simulink model "torque_control_model_7"  (R2018b)
settings: Solver=VariableStepAuto  StartTime=0.0  StopTime=.5  RelTol=1e-3
PreLoadFcn:
  | BLDC_motor_constants_2;
undefined symbols (not defined in the file or in its folder): sigbuilder_block
libraries: powerlib x13, simulink x2, peBldcCurrentController x1
settings Model: Creator=Zach  LastModifiedBy=Zach

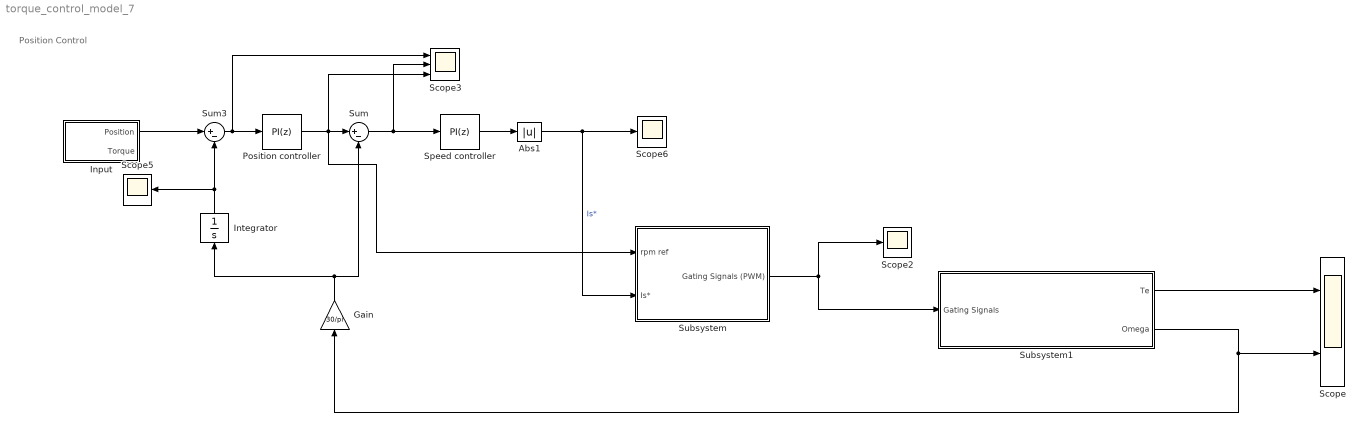
== system torque_control_model_7 ==
  note: Position Control
  Abs1 : Abs
  Gain : Gain  Gain=30/pi
  Input : Subsystem  Tag=STV Subsys  LoadFcn=sigbuilder_block('load');  StartFcn=sigbuilder_block('start');  StopFcn=sigbuilder_block('stop');  ClipboardFcn=sigbuilder_block('clipboard');  mask(Sigbuilder block){tuvar=[0:10]}
      mask help: Simulink:masks:SigbuilderBlock_MD
      mask init:
      | if ~strcmp(get_param(bdroot(gcbh),'SimulationStatus'),'stopped') tuvar = sigbuilder_block('maskInit'); end
      settings: CopyFcn=sigbuilder_block('copy');  DeleteFcn=sigbuilder_block('delete');  ModelCloseFcn=sigbuilder_block('modelClose');  PreSaveFcn=sigbuilder_block('preSave');  PauseFcn=sigbuilder_block('pause');  ContinueFcn=sigbuilder_block('continue');  NameChangeFcn=sigbuilder_block('namechange');  OpenFcn=sigbuilder_block('open',[268.5 149.25 631.5 540 ]);  CloseFcn=sigbuilder_block('close');
      mask Display: plot(0, 0, 100, 100,[2, 2, 32, 32, 2], [68, 8, 8, 68, 68],[32, 2], [38, 38], [32, 19, 2],[53, 60, 44], [32, 17, 17, 2],[16, 16, 31, 31]);txt = getActiveGroup(gcbh);text(2, 100, txt,'verticalAlignment', 'top');
  Integrator : Integrator
  Position controller : simulink/Continuous/PID Controller  Controller=PI  Form=Parallel  TimeDomain=Discrete-time  SampleTime=-1  IntegratorMethod=Forward Euler  FilterMethod=Forward Euler  ControllerParametersSource=internal  P=80  I=5  D=0.5  UseFilter=on  N=100  TunerSelectOption=Transfer Function Based (PID Tuner App)  InitialConditionSource=internal  InitialConditionForIntegrator=0  InitialConditionForFilter=0  DifferentiatorICPrevScaledInput=0  ExternalReset=none  TrackingMode=off  Kt=1  LimitOutput=off  UpperSaturationLimit=10000  LowerSaturationLimit=-10000  LinearizeAsGain=on  AntiWindupMode=back-calculation  Kb=100  POutMin=[]  POutMax=[]  IOutMin=[]  IOutMax=[]  DOutMin=[]  DOutMax=[]  NOutMin=[]  NOutMax=[]  SumOutMin=[]  SumOutMax=[]  SaturationOutMin=[]  SaturationOutMax=[]  PParamMin=[]  PParamMax=[]  IParamMin=[]  IParamMax=[]  DParamMin=[]  DParamMax=[]  NParamMin=[]  NParamMax=[]  KbParamMin=[]  KbParamMax=[]  KtParamMin=[]  KtParamMax=[]  KbOutMin=[]  KbOutMax=[]  KtOutMin=[]  KtOutMax=[]  IntegratorOutMin=[]  IntegratorOutMax=[]  FilterOutMin=[]  FilterOutMax=[]  SumI1OutMin=[]  SumI1OutMax=[]  SumI2OutMin=[]  SumI2OutMax=[]  SumI3OutMin=[]  SumI3OutMax=[]  SumI4OutMin=[]  SumI4OutMax=[]  SumDOutMin=[]  SumDOutMax=[]  DifferentiatorOutMin=[]  DifferentiatorOutMax=[]  FilterDiffOutCoefMin=[]  FilterDiffOutCoefMax=[]  ReciprocalOutMin=[]  ReciprocalOutMax=[]  SumDenOutMin=[]  SumDenOutMax=[]  SumNumOutMin=[]  SumNumOutMax=[]  DivideOutMin=[]  DivideOutMax=[]  IntegratorContinuousStateAttributes=''  IntegratorStateMustResolveToSignalObject=off  IntegratorRTWStateStorageClass=Auto  FilterContinuousStateAttributes=''  FilterStateMustResolveToSignalObject=off  FilterRTWStateStorageClass=Auto  ParallelPVariant=InternalParameters  IdealPVariant=Disabled  IVariant=InternalParameters  DVariant=Disabled  IntegratorVariant=Discrete  SatVariant=Disabled  AWVariant=Passthrough  PCopyVariant=Disabled  TRVariant=Disabled  FdbkBlocksVariant=Forward  IdealPFdbkVariant=Disabled  SatFdbkVariant=Disabled  DerivativeFilterVariant=Disabled  NVariant=Disabled  NCopyVariant=Disabled_SignalSpec  FilterICVariant=Disabled  IntegratorICVariant=InternalICs  ExternalResetVariant=Disabled  TRSumVariant=Passthrough  SumFdbkVariant=Disabled  SumVariant=Sum_PI
  Scope : Scope  NumInputPorts=2
  Scope2 : Scope
  Scope3 : Scope  NumInputPorts=3
  Scope5 : Scope
  Scope6 : Scope
  Speed controller : simulink/Continuous/PID Controller  Controller=PI  Form=Parallel  TimeDomain=Discrete-time  SampleTime=-1  IntegratorMethod=Forward Euler  FilterMethod=Forward Euler  ControllerParametersSource=internal  P=.01  I=15  D=0.5  UseFilter=on  N=100  TunerSelectOption=Transfer Function Based (PID Tuner App)  InitialConditionSource=internal  InitialConditionForIntegrator=0  InitialConditionForFilter=0  DifferentiatorICPrevScaledInput=0  ExternalReset=none  TrackingMode=off  Kt=1  LimitOutput=on  UpperSaturationLimit=500  LowerSaturationLimit=-500  LinearizeAsGain=on  AntiWindupMode=back-calculation  Kb=100  POutMin=[]  POutMax=[]  IOutMin=[]  IOutMax=[]  DOutMin=[]  DOutMax=[]  NOutMin=[]  NOutMax=[]  SumOutMin=[]  SumOutMax=[]  SaturationOutMin=[]  SaturationOutMax=[]  PParamMin=[]  PParamMax=[]  IParamMin=[]  IParamMax=[]  DParamMin=[]  DParamMax=[]  NParamMin=[]  NParamMax=[]  KbParamMin=[]  KbParamMax=[]  KtParamMin=[]  KtParamMax=[]  KbOutMin=[]  KbOutMax=[]  KtOutMin=[]  KtOutMax=[]  IntegratorOutMin=[]  IntegratorOutMax=[]  FilterOutMin=[]  FilterOutMax=[]  SumI1OutMin=[]  SumI1OutMax=[]  SumI2OutMin=[]  SumI2OutMax=[]  SumI3OutMin=[]  SumI3OutMax=[]  SumI4OutMin=[]  SumI4OutMax=[]  SumDOutMin=[]  SumDOutMax=[]  DifferentiatorOutMin=[]  DifferentiatorOutMax=[]  FilterDiffOutCoefMin=[]  FilterDiffOutCoefMax=[]  ReciprocalOutMin=[]  ReciprocalOutMax=[]  SumDenOutMin=[]  SumDenOutMax=[]  SumNumOutMin=[]  SumNumOutMax=[]  DivideOutMin=[]  DivideOutMax=[]  IntegratorContinuousStateAttributes=''  IntegratorStateMustResolveToSignalObject=off  IntegratorRTWStateStorageClass=Auto  FilterContinuousStateAttributes=''  FilterStateMustResolveToSignalObject=off  FilterRTWStateStorageClass=Auto  ParallelPVariant=InternalParameters  IdealPVariant=Disabled  IVariant=InternalParameters  DVariant=Disabled  IntegratorVariant=Discrete  SatVariant=Enabled  AWVariant=BackCalculation  PCopyVariant=Disabled  TRVariant=Disabled  FdbkBlocksVariant=Forward  IdealPFdbkVariant=Disabled  SatFdbkVariant=Disabled  DerivativeFilterVariant=Disabled  NVariant=Disabled  NCopyVariant=Disabled_SignalSpec  FilterICVariant=Disabled  IntegratorICVariant=InternalICs  ExternalResetVariant=Disabled  TRSumVariant=Passthrough  SumFdbkVariant=Disabled  SumVariant=Sum_PI
  Subsystem : Subsystem
  Subsystem1 : Subsystem
  Sum : Sum  Inputs=|+-
  Sum3 : Sum  Inputs=|+-
  wires:
  Subsystem1/1(Te) -> Scope/1
  Position controller/1 -> Subsystem/1(rpm ref), Sum/1, Scope3/3
  Speed controller/1 -> Abs1/1
  Sum/1 -> Scope3/2, Speed controller/1
  Subsystem1/2(Omega) -> Scope/2, Gain/1
  Sum3/1 -> Scope3/1, Position controller/1
  Integrator/1 -> Sum3/2, Scope5/1
  Input/1(Position) -> Sum3/1
  Abs1/1 -> Scope6/1, Subsystem/2(Is*)  "Is*"
  Gain/1 -> Integrator/1, Sum/2
  Subsystem/1(Gating Signals (PWM)) -> Subsystem1/1(Gating Signals), Scope2/1

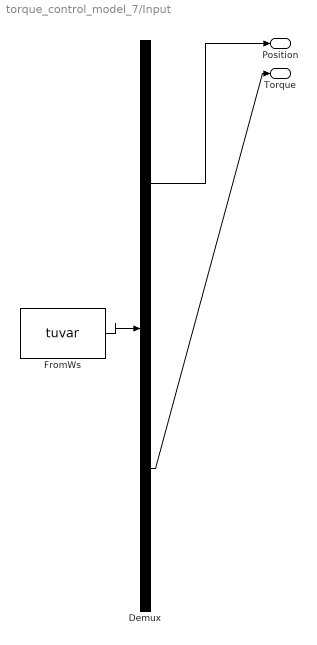
== system torque_control_model_7/Input ==
  Demux : Demux  Tag=STV Demux  Outputs=2
  FromWs : FromWorkspace  Tag=STV FromWs  VariableName=tuvar  SampleTime=0
      SigBuilderData=|
      | common.afterFinalStr = 'Extrapolate'
      | common.sampleTime = 0
      | dataSet.timeRange = [0 2]
      | dataSet.name = 'Test 1'
      | sbobj.Groups.Name = 'Test 1'
      | sbobj.Groups.Signals(1).Name = 'Position'
      | sbobj.Groups.Signals(1).XData = [0 0.1 0.1 0.805 0.805 1.405 1.405 2]
      | sbobj.Groups.Signals(1).YData = [0 1 80 80 100 100 20 20]
      | sbobj.Groups.Signals(2).Name = 'Torque'
      | sbobj.Groups.Signals(2).XData = [0 0.5 0.5 2]
      | sbobj.Groups.Signals(2).YData = [0 0 3 3]
      | sbobj.Groups.TimeRange = [0 2]
  Position : Outport  Tag=STV Outport
  Torque : Outport  Tag=STV Outport  Port=2
  wires:
  FromWs/1 -> Demux/1
  Demux/1 -> Position/1
  Demux/2 -> Torque/1

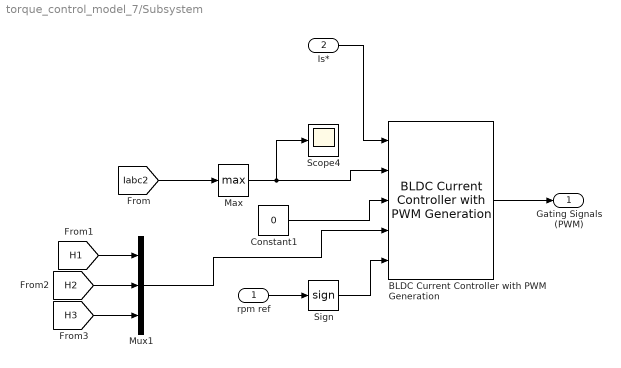
== system torque_control_model_7/Subsystem ==
  rpm ref : Inport
  Is* : Inport  Port=2
  BLDC Current Controller with PWM Generation : peBldcCurrentController/BLDC Current Controller with PWM Generation  Kp=40  Ki=1  Kaw=100  Ts=-1  Tsd=0.001  ActZC=off  CarrCount=Up  Tper=.0001  Tfundamental=.00001
  Constant1 : Constant  Value=0
  Max : MinMax  Function=max
  Mux1 : Mux  Inputs=3
  Scope4 : Scope
  Sign : Signum
  Gating Signals (PWM) : Outport
  wires:
  rpm ref/1 -> Sign/1
  Mux1/1 -> BLDC Current Controller with PWM Generation/4
  [Iabc2] -> Max/1
  [H1] -> Mux1/1
  [H3] -> Mux1/3
  Sign/1 -> BLDC Current Controller with PWM Generation/5
  Constant1/1 -> BLDC Current Controller with PWM Generation/3
  Max/1 -> BLDC Current Controller with PWM Generation/2, Scope4/1
  [H2] -> Mux1/2
  BLDC Current Controller with PWM Generation/1 -> Gating Signals (PWM)/1
  Is*/1 -> BLDC Current Controller with PWM Generation/1

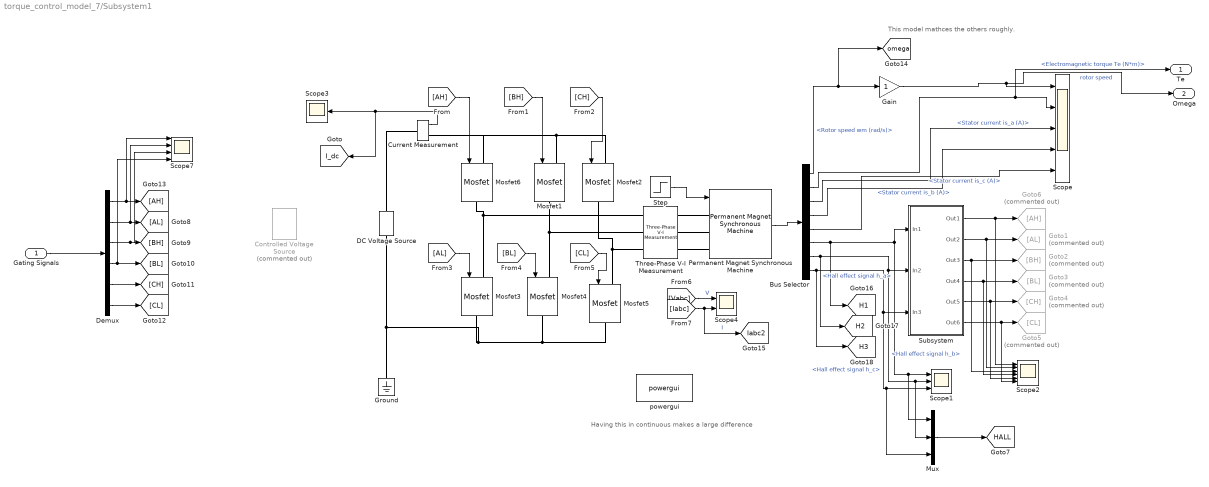
== system torque_control_model_7/Subsystem1 ==
  note: This model mathces the others roughly.
  note: Having this in continuous makes a large difference
  Gating Signals : Inport
  Bus Selector : BusSelector  OutputSignals=Rotor speed wm (rad/s),Electromagnetic torque Te (N*m),Stator current is_a (A),Stator current is_b (A),Stator current is_c (A),Hall effect signal h_a,Hall effect signal h_b,Hall effect signal h_c
  Controlled Voltage Source : powerlib/Electrical Sources/Controlled Voltage Source  Commented=on  Initialize=off  Source_Type=DC  Amplitude=24  Phase=0  Frequency=0  Measurements=Voltage
  Current Measurement : powerlib/Measurements/Current Measurement  PhasorSimulation=off  OutputType=Magnitude  PSBequivalent=0
  DC Voltage Source : powerlib/Electrical Sources/DC Voltage Source  Amplitude=24  Measurements=None
  Demux : Demux  Outputs=6
  Gain : Gain
  Goto1 : Goto  Commented=on  GotoTag=AL
  Goto2 : Goto  Commented=on  GotoTag=BH
  Goto3 : Goto  Commented=on  GotoTag=BL
  Goto4 : Goto  Commented=on  GotoTag=CH
  Goto5 : Goto  Commented=on  GotoTag=CL
  Goto6 : Goto  Commented=on  GotoTag=AH
  Ground : powerlib/Elements/Ground  LConnTagsString=a
  Mosfet{1..6} (6 alike) : powerlib/Power Electronics/Mosfet  Ron=0.1  Lon=0  Rd=0.01  Vfd=0  IC=0  Rs=1e5  Cs=inf  Measurements=off
  Mux : Mux  Inputs=3
  Permanent Magnet Synchronous Machine : powerlib/Machines/Permanent Magnet Synchronous Machine  NbPhases=3  FluxDistribution=Trapezoidal  RotorType=Round  MechanicalLoad=Torque Tm  PresetModel=No  ShowDetailedParameters=on  MeasurementBus=off  Resistance=0.304  Inductance=0.0002315  dqInductances=[8.5e-3,8.5e-3]  La=0.0002315  MachineConstant=Torque Constant (N.m / A_peak)  Flux=0.003258  VoltageCst=5.4588  TorqueCst=0.052128  Flat=120  Mechanical=[1.81e-05 1e-07 8]  PolePairs=4  InitialConditions=[0,0, 0,0]  InitialConditions5ph=[0 0 0 0 0 0]  TsPowergui=0  TsBlock=-1  RefAngle=Aligned with phase A axis (original Park)
      settings: SourceProductName=Simscape Power Systems
  Scope : Scope  NumInputPorts=5
  Scope1 : Scope  NumInputPorts=3
  Scope2 : Scope  NumInputPorts=6
  Scope3 : Scope
  Scope4 : Scope  NumInputPorts=2
  Scope7 : Scope  NumInputPorts=4
  Step : Step  Time=.08  After=.02  SampleTime=0
  Subsystem : Subsystem
  Three-Phase V-I Measurement : powerlib/Measurements/Three-Phase V-I Measurement  VoltageMeasurement=phase-to-ground  SetLabelV=on  LabelV=Vabc  Vpu=off  VpuLL=off  CurrentMeasurement=yes  SetLabelI=on  LabelI=Iabc  Ipu=off  Pbase=100e6  Vbase=500e3  OutputType=Complex  PhasorSimulation=off  PSBequivalent=0
  powergui : powerlib/powergui  Priority=1  SimulationMode=Continuous  SampleTime=50e-6  frequency=60  Iterations=50  frequencyindice=0  Pbase=100e6  ErrMax=1e-4  UnitsV=kV  UnitsW=MW  buscounter=0  FunctionMessages=off  echomessages=off  EnableUseOfTLC=off  CurrentSourceSwitches=off  DisableSnubberDevices=off  DisableRonSwitches=off  DisableVfSwitches=off  DisplayEquations=off  SolverType=Tustin/Backward Euler (TBE)  Interpol=off  ExternalGateDelay=off  methode=off  Ts=100  x0status=blocks  SPID=on  SwTol=0  HookPort=off  RestoreLinks=warning  ResistiveCurrentMeasurement=off  Frange=[0:2:500]  Ylog=off  Xlog=on  ShowGrid=off  save=off  variable=ZData  structure=0  ZoomFFT=off  StartTime=0.0  cycles=1  DisplayStyle=1  fundamental=60  FreqAxis=off  MaxFrequency=1000  frequencyindicesteady=1  RmsSteady=1  display=off
  Te : Outport
  Omega : Outport  Port=2
  tag scope: H1=global, H2=global, H3=global, HALL=global, I_dc=global, Iabc2=global, omega=global
  wires:
  [CH] -> Mosfet2/1
  Subsystem/6(Out6) -> Scope2/6, Goto5/1
  Subsystem/2(Out2) -> Scope2/2, Goto1/1
  Bus Selector/8 -> [H3], Mux/3, Scope1/3, Subsystem/3(In3)  "<Hall effect signal h_c>"
  Subsystem/1(Out1) -> Scope2/1, Goto6/1
  Subsystem/3(Out3) -> Scope2/3, Goto2/1
  Bus Selector/2 -> Te/1, Scope/2  "<Electromagnetic torque Te (N*m)>"
  Subsystem/4(Out4) -> Scope2/4, Goto3/1
  Bus Selector/1 -> [omega], Gain/1  "<Rotor speed wm (rad/s)>"
  Bus Selector/7 -> [H2], Mux/2, Scope1/2, Subsystem/2(In2)  "<Hall effect signal h_b>"
  Mux/1 -> [HALL]
  [AL] -> Mosfet3/1
  [BL] -> Mosfet4/1
  Bus Selector/6 -> [H1], Subsystem/1(In1), Mux/1, Scope1/1  "<Hall effect signal h_a>"
  Subsystem/5(Out5) -> Scope2/5, Goto4/1
  [CL] -> Mosfet5/1
  Current Measurement/1 -> Scope3/1, [I_dc]
  Bus Selector/3 -> Scope/3  "<Stator current is_a (A)>"
  Permanent Magnet Synchronous Machine/1 -> Bus Selector/1
  [BH] -> Mosfet1/1
  [AH] -> Mosfet6/1
  Bus Selector/4 -> Scope/4  "<Stator current is_b (A)>"
  Gain/1 -> Omega/1, Scope/1  "rotor speed"
  Step/1 -> Permanent Magnet Synchronous Machine/1
  Bus Selector/5 -> Scope/5  "<Stator current is_c (A)>"
  Demux/6 -> [CL]
  Demux/5 -> [CH]
  Demux/4 -> [BL], Scope7/4
  Demux/3 -> Scope7/3, [BH]
  Demux/2 -> Scope7/2, [AL]
  Demux/1 -> Scope7/1, [AH]
  [Vabc] -> Scope4/1  "V"
  [Iabc] -> [Iabc2], Scope4/2  "I"
  Gating Signals/1 -> Demux/1
  connections:
  Mosfet1/RConn1 -- Three-Phase V-I Measurement/LConn2 -- Mosfet4/LConn1
  Mosfet2/RConn1 -- Three-Phase V-I Measurement/LConn3 -- Mosfet5/LConn1
  Mosfet6/RConn1 -- Three-Phase V-I Measurement/LConn1 -- Mosfet3/LConn1
  Mosfet6/LConn1 -- Current Measurement/RConn1 -- Mosfet2/LConn1 -- Mosfet1/LConn1
  Ground/LConn1 -- DC Voltage Source/LConn1 -- Mosfet5/RConn1 -- Mosfet4/RConn1 -- Mosfet3/RConn1
  Three-Phase V-I Measurement/RConn1 -- Permanent Magnet Synchronous Machine/LConn1
  Three-Phase V-I Measurement/RConn2 -- Permanent Magnet Synchronous Machine/LConn2
  Permanent Magnet Synchronous Machine/LConn3 -- Three-Phase V-I Measurement/RConn3
  DC Voltage Source/RConn1 -- Current Measurement/LConn1

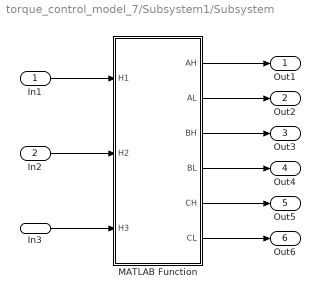
== system torque_control_model_7/Subsystem1/Subsystem ==
  In1 : Inport
  In2 : Inport  Port=2
  In3 : Inport  Port=3
  MATLAB Function : MATLAB Function  TreatAsAtomicUnit=on
  Out1 : Outport
  Out2 : Outport  Port=2
  Out3 : Outport  Port=3
  Out4 : Outport  Port=4
  Out5 : Outport  Port=5
  Out6 : Outport  Port=6
  wires:
  In1/1 -> MATLAB Function/1(H1)
  In3/1 -> MATLAB Function/3(H3)
  In2/1 -> MATLAB Function/2(H2)
  MATLAB Function/1(AH) -> Out1/1
  MATLAB Function/2(AL) -> Out2/1
  MATLAB Function/3(BH) -> Out3/1
  MATLAB Function/4(BL) -> Out4/1
  MATLAB Function/6(CL) -> Out6/1
  MATLAB Function/5(CH) -> Out5/1

== matlab function torque_control_model_7/Subsystem1/Subsystem/MATLAB Function ==
  data: H1 input; AH output; H2 input; H3 input; AL output; BH output; BL output; CH output; CL output
function [AH, AL, BH, BL, CH, CL] = fcn(H1, H2, H3)
% H1 = int16(H1);
% H2 = int16(H2);
% H3 = int16(H3);
H1
H2
H3
AH = 0;
AL = 0;
BH = 0;
BL = 0;
CH = 0;
CL = 0;
%Rember this does not deal with the PWM signal
if (H1(1) == 1 && H2 == 0 && H3 == 0)
    AH = 1;
    AL = 0;
    BH = 0;
    BL = 1;
    CH = 0;
    CL = 0;
elseif (H1(1) == 1 && H2 == 1 && H3 == 0)
    AH = 1;
    AL = 0;
    BH = 0;
    BL = 0;
    CH = 0;
    CL = 1;
elseif (H1(1) == 0 && H2 == 1 && H3 == 0)
    AH = 0;
    AL = 0;
    BH = 1;
    BL = 0;
    CH = 0;
    CL = 1;
elseif (H1(1) == 0 && H2 == 1 && H3 == 1)
    AH = 0;
    AL = 1;
    BH = 1;
    BL = 0;
    CH = 0;
    CL = 0;
elseif (H1(1) == 0 && H2 == 0 && H3 == 1)
    AH = 0;
    AL = 1;
    BH = 0;
    BL = 0;
    CH = 1;
    CL = 0;
elseif (H1(1) == 1 && H2 == 0 && H3 == 1)
    AH = 0;
    AL = 0;
    BH = 0;
    BL = 1;
    CH = 1;
    CL = 0;
end
